simulink model "Simulink_APP4S5"  (R2019a)
settings: Solver=ode45  StartTime=0.0  StopTime=5  RelTol=1e-3
values from neighbouring files (symbols this model uses):
  A = [0,         v,      0 ... (first row only)    [loadAutoPilotLinearMatrices.m]    (also in loadParkingLinearMatrices.m = [0,         0,      0)
  Asim = 0.01    [loadconstants.m]
  B = [0,         0 ... (first row only)    [loadAutoPilotLinearMatrices.m]    (also in loadParkingLinearMatrices.m = [1,         0)
  bm = 0.00001    (= 1e-05)    [loadconstants.m]
  C = [0, 0, 1 ... (first row only)    [loadAutoPilotLinearMatrices.m]    (also in loadParkingLinearMatrices.m = [1, 0, 0)
  Cd = 0.5    [loadconstants.m]
  Cr = 0.01    [loadconstants.m]
  D = [0, 0 ... (first row only)    [loadAutoPilotLinearMatrices.m]    (also in loadParkingLinearMatrices.m)
  g = 9.81    [loadconstants.m]
  Jm = 0.00005    (= 5e-05)    [loadconstants.m]
  Km = 0.0028    [loadconstants.m]
  Lm = 0.0001    [loadconstants.m]
  m = 5    [loadconstants.m]
  N = -inv(C*inv(A-(B*KautoPilot))*B)    [app.m]    (also in loadAutoPilotCostMatrices.m = 0)
  Nsim = 15.3    [loadconstants.m]
  rho = 1.204    [loadconstants.m]
  Rm = 0.64    [loadconstants.m]
  rsim = 0.04    [loadconstants.m]
  speedReference = 2    [loadconstants.m]
  Ts = 0.01    [loadconstants.m]
  x0 = [0 ... (first row only)    [loadconstants.m]
  yReferenceAuto = 0    [loadconstants.m]
undefined symbols (not defined in the file or in its folder): Continuous, KautoPilot, sigbuilder_block, Time
libraries: simulink x4, ctrlSharedLib x1
settings Model: Creator=samuel  LastModifiedBy=samuel
settings SolverCC: ZeroCrossAlgorithm=Adaptive
settings DebuggingCC: IgnoredZcDiagnostic=none

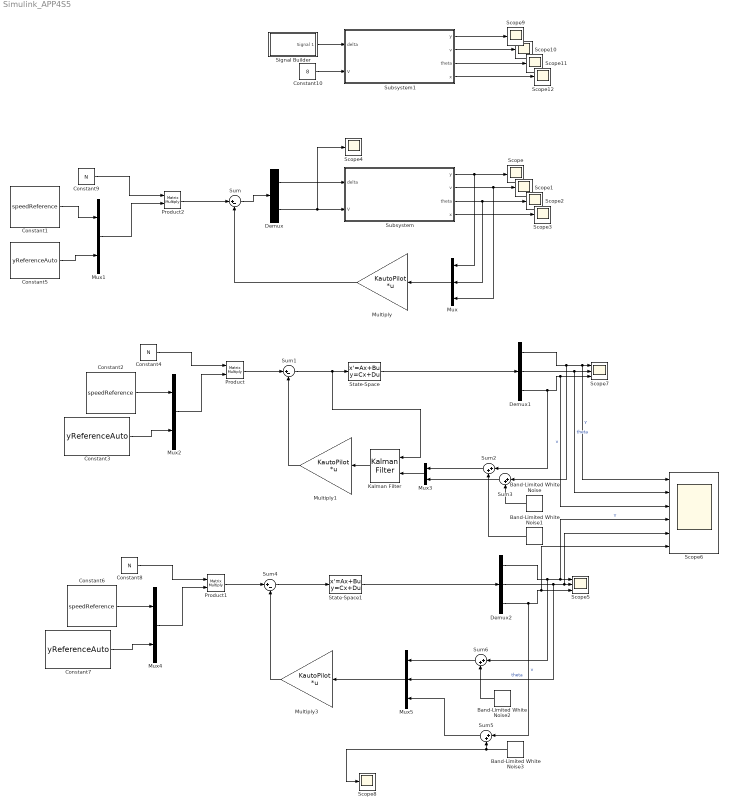
== system Simulink_APP4S5 ==
  Band-Limited White Noise : simulink/Sources/Band-Limited White Noise  Cov=[0.00001]  Ts=0.1  seed=[23341]
  Band-Limited White Noise1 : simulink/Sources/Band-Limited White Noise  Cov=[0.00001]  Ts=0.1  seed=[23341]
  Band-Limited White Noise2 : simulink/Sources/Band-Limited White Noise  Cov=[0.0001]  Ts=0.1  seed=[23341]
  Band-Limited White Noise3 : simulink/Sources/Band-Limited White Noise  Cov=[0.005]  Ts=0.1  seed=[23341]
  Constant1 : Constant  Value=speedReference
  Constant10 : Constant  Value=8
  Constant2 : Constant  Value=speedReference
  Constant3 : Constant  Value=yReferenceAuto
  Constant4 : Constant  Value=N
  Constant5 : Constant  Value=yReferenceAuto
  Constant6 : Constant  Value=speedReference
  Constant7 : Constant  Value=yReferenceAuto
  Constant8 : Constant  Value=N
  Constant9 : Constant  Value=N
  Demux : Demux  Outputs=2
  Demux1 : Demux  Outputs=3
  Demux2 : Demux  Outputs=3
  Kalman Filter : ctrlSharedLib/Kalman Filter  TimeDomain=Continuous-Time  UseCurrentEstimator=on  ModelSource=Individual A, B, C, D matrices  ModelSourceVariable=ss(0.95,1,1,0,1)  A=A  B=B  C=C  D=D  NumberOfStates=1  NumberOfInputs=1  NumberOfOutputs=1  InitialEstimateSource=Dialog  X0=x0  P0=10  UseK=off  UseGH=off  NumberOfProcessNoiseInputs=1  G=1  TimeInvariantG=on  H=0  TimeInvariantH=on  Q=0.05  TimeInvariantQ=on  R=1  TimeInvariantR=on  N=0  TimeInvariantN=on  AddInputPort=on  AddEnablePort=off  OutputEstimatedY=off  OutputP=off  Ts=-1
      settings: SourceProductBaseCode=CT
  Multiply : Gain  Gain=KautoPilot  Multiplication=Matrix(K*u) (u vector)
  Multiply1 : Gain  Gain=KautoPilot  Multiplication=Matrix(K*u) (u vector)
  Multiply3 : Gain  Gain=KautoPilot  Multiplication=Matrix(K*u) (u vector)
  Mux : Mux  Inputs=3
  Mux{1..4} (4 alike) : Mux  Inputs=2
  Mux5 : Mux  Inputs=3
  Product : Product  Multiplication=Matrix(*)
  Product1 : Product  Multiplication=Matrix(*)
  Product2 : Product  Multiplication=Matrix(*)
  Scope{,1..4,8..12} (10 alike) : Scope
  Scope5 : Scope  NumInputPorts=3
  Scope6 : Scope  NumInputPorts=6
  Scope7 : Scope  NumInputPorts=3
  Signal Builder : Subsystem  Tag=STV Subsys  LoadFcn=sigbuilder_block('load');  StartFcn=sigbuilder_block('start');  StopFcn=sigbuilder_block('stop');  ClipboardFcn=sigbuilder_block('clipboard');  mask(Sigbuilder block){tuvar=[0:10]}
      mask help: Simulink:masks:SigbuilderBlock_MD
      mask init:
      | if ~strcmp(get_param(bdroot(gcbh),'SimulationStatus'),'stopped') tuvar = sigbuilder_block('maskInit'); end
      settings: CopyFcn=sigbuilder_block('copy');  DeleteFcn=sigbuilder_block('delete');  ModelCloseFcn=sigbuilder_block('modelClose');  PreSaveFcn=sigbuilder_block('preSave');  PauseFcn=sigbuilder_block('pause');  ContinueFcn=sigbuilder_block('continue');  NameChangeFcn=sigbuilder_block('namechange');  OpenFcn=sigbuilder_block('open',[433.5 195.75 558 394.5 ]);  CloseFcn=sigbuilder_block('close');
      mask Display: plot(0, 0, 100, 100,[2, 2, 32, 32, 2], [68, 8, 8, 68, 68],[32, 2], [38, 38], [32, 19, 2],[53, 60, 44], [32, 17, 17, 2],[16, 16, 31, 31]);txt = getActiveGroup(gcbh);text(2, 100, txt,'verticalAlignment', 'top');
  State-Space : StateSpace  A=A  B=B  C=[1 0 0; 0 1 0; 0 0 1]  D=[0 0; 0 0; 0 0]  InitialCondition=x0
  State-Space1 : StateSpace  A=A  B=B  C=[1 0 0; 0 1 0; 0 0 1]  D=[0 0; 0 0; 0 0]  InitialCondition=x0
  Subsystem : Subsystem
  Subsystem1 : Subsystem
  Sum : Sum  Inputs=|+-
  Sum1 : Sum  Inputs=|+-
  Sum{2..3,5..6} (4 alike) : Sum  Inputs=|++
  Sum4 : Sum  Inputs=|+-
  wires:
  Subsystem/1(y) -> Mux/1, Scope/1
  Subsystem/2("v ") -> Mux/3, Scope1/1
  Subsystem/3("theta ") -> Mux/2, Scope2/1
  Subsystem/4(x) -> Scope3/1
  Mux/1 -> Multiply/1
  Demux/1 -> Subsystem/1(delta)
  Demux/2 -> Scope4/1, Subsystem/2(V)
  State-Space/1 -> Demux1/1
  Sum1/1 -> Kalman Filter/1, State-Space/1
  Constant2/1 -> Mux2/1
  Constant3/1 -> Mux2/2
  Multiply1/1 -> Sum1/2
  Demux1/1 -> Sum3/1, Scope6/1, Scope7/1  "Y"
  Demux1/2 -> Scope6/2, Scope7/2  "theta"
  Demux1/3 -> Sum2/1, Scope6/3, Scope7/3  "v"
  Product/1 -> Sum1/1
  Constant4/1 -> Product/1
  Mux2/1 -> Product/2
  Constant5/1 -> Mux1/2
  Constant1/1 -> Mux1/1
  Multiply/1 -> Sum/2
  Sum/1 -> Demux/1
  Kalman Filter/1 -> Multiply1/1
  Mux3/1 -> Kalman Filter/2
  Sum2/1 -> Mux3/1
  Sum3/1 -> Mux3/2
  Band-Limited White Noise/1 -> Sum3/2
  Band-Limited White Noise1/1 -> Sum2/2
  State-Space1/1 -> Demux2/1
  Demux2/1 -> Sum6/1, Scope6/4, Scope5/1  "Y"
  Constant8/1 -> Product1/1
  Mux4/1 -> Product1/2
  Constant6/1 -> Mux4/1
  Band-Limited White Noise3/1 -> Scope8/1, Sum5/2
  Sum4/1 -> State-Space1/1
  Constant7/1 -> Mux4/2
  Demux2/2 -> Mux5/2, Scope6/5, Scope5/2  "theta"
  Band-Limited White Noise2/1 -> Sum6/2
  Product1/1 -> Sum4/1
  Multiply3/1 -> Sum4/2
  Demux2/3 -> Sum5/1, Scope6/6, Scope5/3  "v"
  Mux5/1 -> Multiply3/1
  Sum6/1 -> Mux5/1
  Sum5/1 -> Mux5/3
  Constant9/1 -> Product2/1
  Mux1/1 -> Product2/2
  Product2/1 -> Sum/1
  Subsystem1/2("v ") -> Scope10/1
  Subsystem1/4(x) -> Scope12/1
  Subsystem1/1(y) -> Scope9/1
  Constant10/1 -> Subsystem1/2(V)
  Signal Builder/1(Signal 1) -> Subsystem1/1(delta)
  Subsystem1/3("theta ") -> Scope11/1

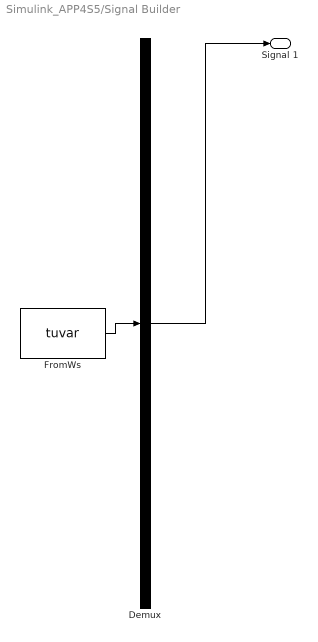
== system Simulink_APP4S5/Signal Builder ==
  Demux : Demux  Tag=STV Demux  Outputs=1
  FromWs : FromWorkspace  Tag=STV FromWs  VariableName=tuvar  SampleTime=0
      SigBuilderData=|
      | common.afterFinalStr = 'Extrapolate'
      | common.sampleTime = 0
      | dataSet.timeRange = [0 10]
      | dataSet.name = 'Group 1'
      | sbobj.Groups.Name = 'Group 1'
      | sbobj.Groups.Signals.Name = 'Signal 1'
      | sbobj.Groups.Signals.XData = [0 2 2 4 4 10]
      | sbobj.Groups.Signals.YData = [0 0 1 1 0 0]
  Signal 1 : Outport  Tag=STV Outport
  wires:
  Demux/1 -> Signal 1/1
  FromWs/1 -> Demux/1

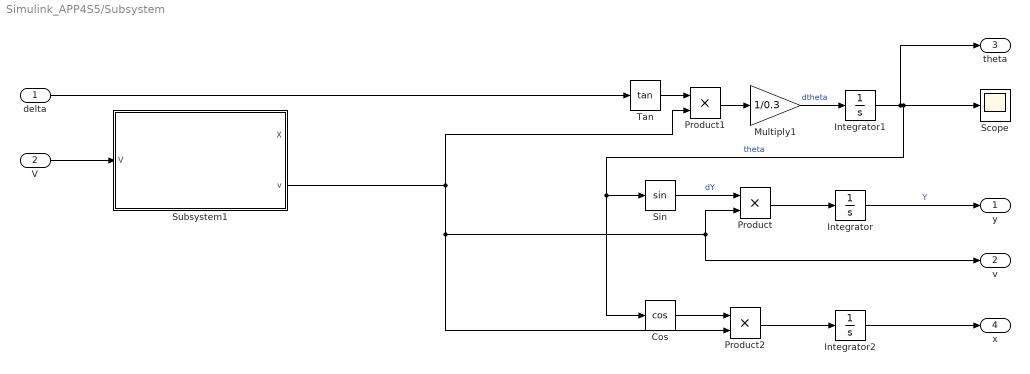
== system Simulink_APP4S5/Subsystem ==
  delta : Inport
  V : Inport  Port=2
  Cos : Trigonometry  Operator=cos
  Integrator : Integrator
  Integrator1 : Integrator
  Integrator2 : Integrator
  Multiply1 : Gain  Gain=1/0.3
  Product : Product
  Product1 : Product
  Product2 : Product
  Scope : Scope
  Sin : Trigonometry
  Subsystem1 : Subsystem
  Tan : Trigonometry  Operator=tan
  y : Outport
  "v " : Outport  Port=2
  "theta " : Outport  Port=3
  x : Outport  Port=4
  wires:
  Tan/1 -> Product1/1
  V/1 -> Subsystem1/1(V)
  Product1/1 -> Multiply1/1
  delta/1 -> Tan/1
  Multiply1/1 -> Integrator1/1  "dtheta"
  Subsystem1/2(v) -> Product1/2, Product2/2, "v "/1, Product/2
  Product/1 -> Integrator/1
  Sin/1 -> Product/1  "dY"
  Integrator/1 -> y/1  "Y"
  Integrator1/1 -> "theta "/1, Scope/1, Cos/1, Sin/1  "theta"
  Cos/1 -> Product2/1
  Product2/1 -> Integrator2/1
  Integrator2/1 -> x/1

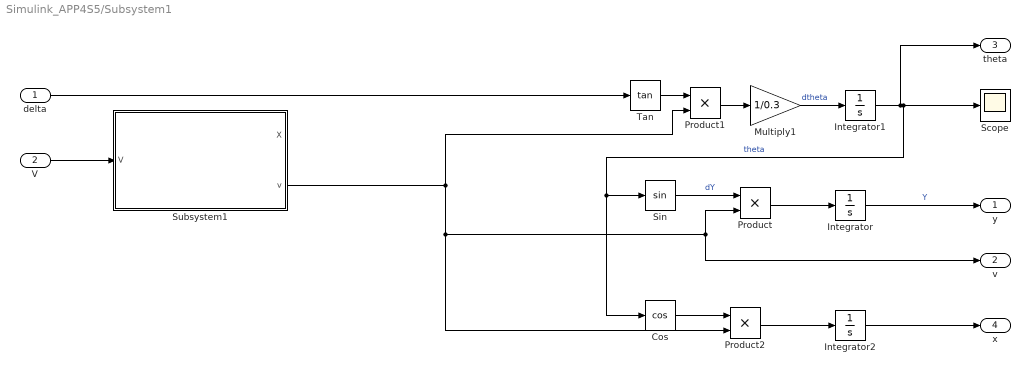
== system Simulink_APP4S5/Subsystem1 ==
  delta : Inport
  V : Inport  Port=2
  Cos : Trigonometry  Operator=cos
  Integrator : Integrator
  Integrator1 : Integrator
  Integrator2 : Integrator
  Multiply1 : Gain  Gain=1/0.3
  Product : Product
  Product1 : Product
  Product2 : Product
  Scope : Scope
  Sin : Trigonometry
  Subsystem1 : Subsystem
  Tan : Trigonometry  Operator=tan
  y : Outport
  "v " : Outport  Port=2
  "theta " : Outport  Port=3
  x : Outport  Port=4
  wires:
  Tan/1 -> Product1/1
  V/1 -> Subsystem1/1(V)
  Product1/1 -> Multiply1/1
  delta/1 -> Tan/1
  Multiply1/1 -> Integrator1/1  "dtheta"
  Subsystem1/2(v) -> Product1/2, Product2/2, "v "/1, Product/2
  Product/1 -> Integrator/1
  Sin/1 -> Product/1  "dY"
  Integrator/1 -> y/1  "Y"
  Integrator1/1 -> "theta "/1, Scope/1, Cos/1, Sin/1  "theta"
  Cos/1 -> Product2/1
  Product2/1 -> Integrator2/1
  Integrator2/1 -> x/1

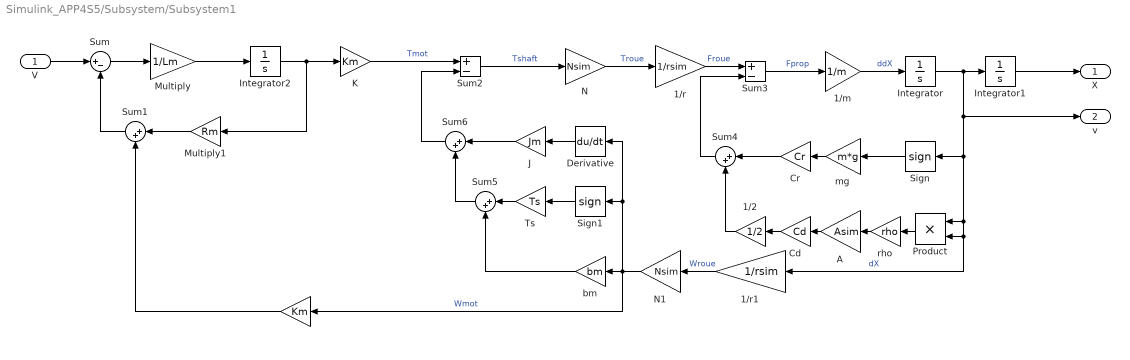
== system Simulink_APP4S5/Subsystem/Subsystem1 ==
  V : Inport
  " " : Gain  Gain=Km
  1/2 : Gain  Gain=1/2
  1/m : Gain  Gain=1/m
  1/r : Gain  Gain=1/rsim
  1/r1 : Gain  Gain=1/rsim
  A : Gain  Gain=Asim
  Cd : Gain  Gain=Cd
  Cr : Gain  Gain=Cr
  Derivative : Derivative
  Integrator : Integrator
  Integrator1 : Integrator
  Integrator2 : Integrator
  J : Gain  Gain=Jm
  K : Gain  Gain=Km
  Multiply : Gain  Gain=1/Lm
  Multiply1 : Gain  Gain=Rm
  N : Gain  Gain=Nsim
  N1 : Gain  Gain=Nsim
  Product : Product
  Sign : Signum  ZeroCross=off
  Sign1 : Signum  ZeroCross=off
  Sum : Sum  Inputs=|+-
  Sum{1,4..6} (4 alike) : Sum  Inputs=|++
  Sum2 : Sum  Inputs=+-
  Sum3 : Sum  Inputs=+-
  Ts : Gain  Gain=Ts
  bm : Gain  Gain=bm
  mg : Gain  Gain=m*g
  rho : Gain  Gain=rho
  X : Outport
  v : Outport  Port=2
  wires:
  Integrator1/1 -> X/1
  rho/1 -> A/1
  Sum2/1 -> N/1  "Tshaft"
  1/m/1 -> Integrator/1  "ddX"
  Product/1 -> rho/1
  1/r1/1 -> N1/1  "Wroue"
  Sum3/1 -> 1/m/1  "Fprop"
  mg/1 -> Cr/1
  N/1 -> 1/r/1  "Troue"
  Sign/1 -> mg/1
  K/1 -> Sum2/1  "Tmot"
  Derivative/1 -> J/1
  A/1 -> Cd/1
  Integrator/1 -> v/1, Product/1, Product/2, 1/r1/1, Sign/1, Integrator1/1  "dX"
  1/r/1 -> Sum3/1  "Froue"
  N1/1 -> Derivative/1, Sign1/1, " "/1, bm/1  "Wmot"
  J/1 -> Sum6/1
  Sum5/1 -> Sum6/2
  bm/1 -> Sum5/2
  Cd/1 -> 1/2/1
  Sum6/1 -> Sum2/2
  Sign1/1 -> Ts/1
  Ts/1 -> Sum5/1
  Sum4/1 -> Sum3/2
  Cr/1 -> Sum4/1
  1/2/1 -> Sum4/2
  Sum/1 -> Multiply/1
  Multiply/1 -> Integrator2/1
  Integrator2/1 -> Multiply1/1, K/1
  Multiply1/1 -> Sum1/1
  " "/1 -> Sum1/2
  V/1 -> Sum/1
  Sum1/1 -> Sum/2

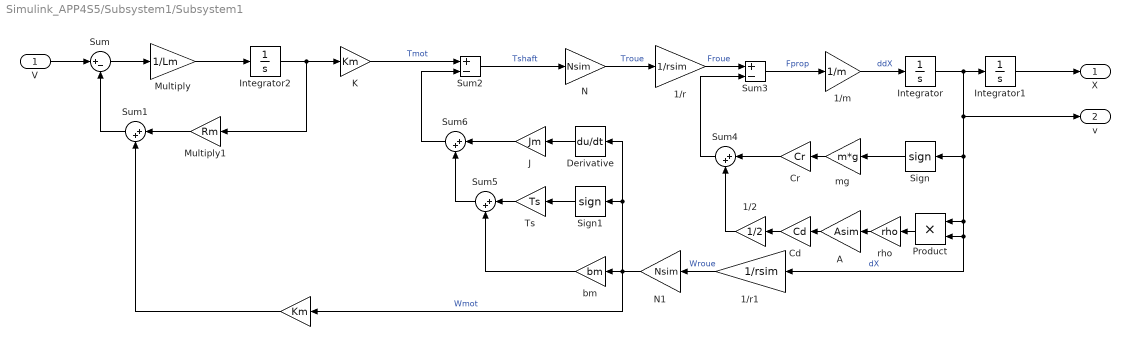
== system Simulink_APP4S5/Subsystem1/Subsystem1 ==
  V : Inport
  " " : Gain  Gain=Km
  1/2 : Gain  Gain=1/2
  1/m : Gain  Gain=1/m
  1/r : Gain  Gain=1/rsim
  1/r1 : Gain  Gain=1/rsim
  A : Gain  Gain=Asim
  Cd : Gain  Gain=Cd
  Cr : Gain  Gain=Cr
  Derivative : Derivative
  Integrator : Integrator
  Integrator1 : Integrator
  Integrator2 : Integrator
  J : Gain  Gain=Jm
  K : Gain  Gain=Km
  Multiply : Gain  Gain=1/Lm
  Multiply1 : Gain  Gain=Rm
  N : Gain  Gain=Nsim
  N1 : Gain  Gain=Nsim
  Product : Product
  Sign : Signum  ZeroCross=off
  Sign1 : Signum  ZeroCross=off
  Sum : Sum  Inputs=|+-
  Sum{1,4..6} (4 alike) : Sum  Inputs=|++
  Sum2 : Sum  Inputs=+-
  Sum3 : Sum  Inputs=+-
  Ts : Gain  Gain=Ts
  bm : Gain  Gain=bm
  mg : Gain  Gain=m*g
  rho : Gain  Gain=rho
  X : Outport
  v : Outport  Port=2
  wires:
  Integrator1/1 -> X/1
  rho/1 -> A/1
  Sum2/1 -> N/1  "Tshaft"
  1/m/1 -> Integrator/1  "ddX"
  Product/1 -> rho/1
  1/r1/1 -> N1/1  "Wroue"
  Sum3/1 -> 1/m/1  "Fprop"
  mg/1 -> Cr/1
  N/1 -> 1/r/1  "Troue"
  Sign/1 -> mg/1
  K/1 -> Sum2/1  "Tmot"
  Derivative/1 -> J/1
  A/1 -> Cd/1
  Integrator/1 -> v/1, Product/1, Product/2, 1/r1/1, Sign/1, Integrator1/1  "dX"
  1/r/1 -> Sum3/1  "Froue"
  N1/1 -> Derivative/1, Sign1/1, " "/1, bm/1  "Wmot"
  J/1 -> Sum6/1
  Sum5/1 -> Sum6/2
  bm/1 -> Sum5/2
  Cd/1 -> 1/2/1
  Sum6/1 -> Sum2/2
  Sign1/1 -> Ts/1
  Ts/1 -> Sum5/1
  Sum4/1 -> Sum3/2
  Cr/1 -> Sum4/1
  1/2/1 -> Sum4/2
  Sum/1 -> Multiply/1
  Multiply/1 -> Integrator2/1
  Integrator2/1 -> Multiply1/1, K/1
  Multiply1/1 -> Sum1/1
  " "/1 -> Sum1/2
  V/1 -> Sum/1
  Sum1/1 -> Sum/2
